simulink model "blovuztb"  (Simulink 8.5)
settings: Solver=ode45  SolverMode=SingleTasking  StartTime=0.0  StopTime=2  RelTol=1e-3  AbsTol=1e-6
settings Model: Creator=PC  LastModifiedBy=PC  ExtModeTrigMode=oneshot  ExtModeArmWhenConnect=off
settings DataIOCC: LimitDataPoints=off
settings OptimizationCC: BlockReduction=off  BooleanDataType=off  ExpressionDepthLimit=128
settings DebuggingCC: SaveWithParameterizedLinksMsg=none  SignalResolutionControl=TryResolveAllWithWarning  MultiTaskDSMMsg=warning  MultiTaskCondExecSysMsg=none  FcnCallInpInsideContextMsg=EnableAllAsError  StateNameClashWarn=none  StrictBusMsg=None
settings HardwareCC: TargetUnknown=on

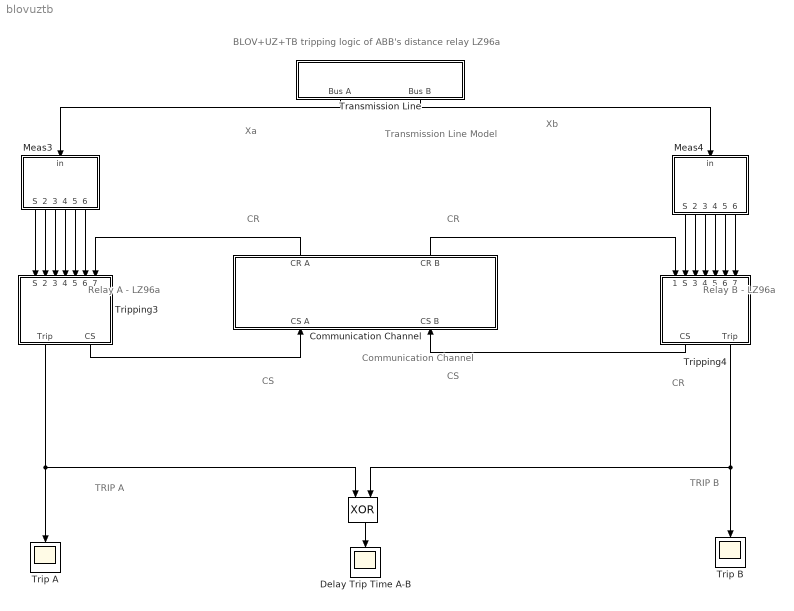
== system blovuztb ==
  note: Relay A - LZ96a
  note: CR
  note: Relay B - LZ96a
  note: Transmission Line Model
  note: Xa
  note: Xb
  note: CS
  note: CS
  note: CR
  note: CR
  note: BLOV+UZ+TB tripping logic of ABB's distance relay LZ96a
  note: Communication
      | Channel
  note: TRIP A
  note: TRIP B
  " " : Logic  Operator=XOR
  Communication Channel : Subsystem  mask(Communication channel.){Tdelay=20, failureA=off, failureB=on, err_signal=1}
      mask prompts: Tdelay "Channel delay time [ms]:"; failureA "A to B Communication channel failure."; failureB "B to A Communication Channel failure"; err_signal "Erroneous signal:"
      mask TypeOptions err_signal: 0 | 1
  Delay Trip Time A-B : Scope
      settings: TickLabels=on  YMin=-0.5  YMax=2
  Meas3 : Subsystem  mask(Tripping Logic){S=[3,1], ZM=[0.8, 1.6, 2.5], t=[0, 0.2, 0.4, 1], ZOV=[1.4, 0.02], ZMB=1.6}
      mask prompts: S "Starter  [Sfore(pu), Sback(pu)]:"; ZM "Zone reach [ZM1(pu), ZM2(pu), ZM3(pu)]:"; t "Zone time [t1(s), t2(s), t3(s), t4(s)] :"; ZOV "[ZOV(pu), tHF(s)] :"; ZMB "ZMB(pu):"
      mask help:
      | ABB LZ96a Distance Relay, BLOV+UZ+TB tripping logic :
      |    starters S (S, Ks, t4)
      |    measuring system M1 (ZM1, ZM2, ZM3), (0, t2, t3)
      |    measuring system M2 (ZOV, tHF)
      |    reverse measurement MB (ZMB)
      mask Help:
      | ABB LZ96a Distance Relay
      | BLOV+UZ+TB tripping logic
      | Blocking overreaching  with independent measuring zone and current reversal logic
  Meas4 : Subsystem  mask(Tripping Logic){S=[3,1], ZM=[0.8, 1.6, 2.5], t=[0, 0.2, 0.4, 1], ZOV=[1.4, 0.02], ZMB=1.6}
      mask prompts: S "Starter  [Sfore(pu), Sback(pu)]:"; ZM "Zone reach [ZM1(pu), ZM2(pu), ZM3(pu)]:"; t "Zone time [t1(s), t2(s), t3(s), t4(s)] :"; ZOV "[ZOV(pu), tHF(s)] :"; ZMB "ZMB(pu):"
      mask help:
      | ABB LZ96a Distance Relay, BLOV+UZ+TB tripping logic :
      |    starters S (S, Ks, t4)
      |    measuring system M1 (ZM1, ZM2, ZM3), (0, t2, t3)
      |    measuring system M2 (ZOV, tHF)
      |    reverse measurement MB (ZMB)
      mask Help:
      | ABB LZ96a Distance Relay
      | BLOV+UZ+TB tripping logic
      | Blocking overreaching  with independent measuring zone and current reversal logic
  Transmission Line : Subsystem  mask(Model of transmission line with fault){x=-0.1, Tfault=0}
      mask prompts: x "Fault location from bus A [p.u.]"; Tfault "Fault time [s]:"
  Trip A : Scope
      settings: TickLabels=on  TimeRange=2  YMin=-0.5  YMax=2
  Trip B : Scope
      settings: TickLabels=on  YMin=-0.5  YMax=2
  Tripping3 : Subsystem
  Tripping4 : Subsystem
  wires:
  Meas3/1(S) -> Tripping3/1(S)
  Meas3/2(ZM1) -> Tripping3/2(ZM1)
  Meas3/3(ZM2) -> Tripping3/3(ZM2)
  Meas3/4(ZM3) -> Tripping3/4(ZM3)
  Meas3/5(ZOV) -> Tripping3/5(ZOV)
  Meas3/6(ZMB) -> Tripping3/6(ZMB)
  Transmission Line/1(Bus A) -> Meas3/1(in)
  Communication Channel/1(CR A) -> Tripping3/7(CR)
  Tripping3/2(CS) -> Communication Channel/1(CS A)
  Meas4/1(S) -> Tripping4/2(S)
  Meas4/2(ZM1) -> Tripping4/3(ZM1)
  Meas4/3(ZM2) -> Tripping4/4(ZM2)
  Meas4/4(ZM3) -> Tripping4/5(ZM3)
  Meas4/5(ZOV) -> Tripping4/6(ZOV)
  Meas4/6(ZMB) -> Tripping4/7(ZMB)
  Transmission Line/2(Bus B) -> Meas4/1(in)
  Tripping4/1(CS) -> Communication Channel/2(CS B)
  Communication Channel/2(CR B) -> Tripping4/1(CR)
  " "/1 -> Delay Trip Time A-B/1
  Tripping3/1(Trip) -> Trip A/1, " "/1
  Tripping4/2(Trip) -> Trip B/1, " "/2

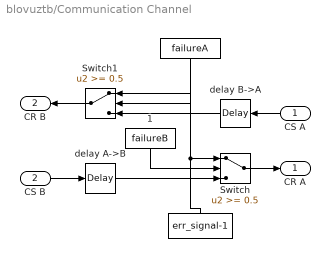
== system blovuztb/Communication Channel ==
  CS A : Inport
  CS B : Inport  Port=2
  " " : Constant  Value=failureA
  "  " : Constant  Value=err_signal-1
  " 1" : Constant  Value=failureB
  Switch : Switch  Threshold=0.5  SaturateOnIntegerOverflow=on  InputSameDT=on
  Switch1 : Switch  Threshold=0.5  SaturateOnIntegerOverflow=on  InputSameDT=on
  delay A->B : TransportDelay  DelayTime=Tdelay/1000+1e-12
  delay B->A : TransportDelay  DelayTime=Tdelay/1000+1e-12
  CR A : Outport  InitialOutput=0
  CR B : Outport  Port=2  InitialOutput=0
  wires:
  Switch/1 -> CR A/1
  CS B/1 -> delay A->B/1
  CS A/1 -> delay B->A/1
  Switch1/1 -> CR B/1
  "  "/1 -> Switch1/1, Switch/1
  delay A->B/1 -> Switch/3
  delay B->A/1 -> Switch1/3
  " "/1 -> Switch1/2
  " 1"/1 -> Switch/2

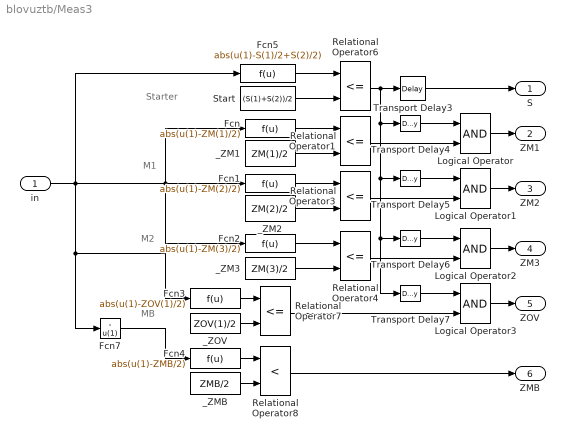
== system blovuztb/Meas3 ==
  note: M1
  note: Starter
  note: M2
  note: MB
  in : Inport
  Fcn : Fcn  Expr=abs(u(1)-ZM(1)/2)
  Fcn1 : Fcn  Expr=abs(u(1)-ZM(2)/2)
  Fcn2 : Fcn  Expr=abs(u(1)-ZM(3)/2)
  Fcn3 : Fcn  Expr=abs(u(1)-ZOV(1)/2)
  Fcn4 : Fcn  Expr=abs(u(1)-ZMB/2)
  Fcn5 : Fcn  Expr=abs(u(1)-S(1)/2+S(2)/2)
  Fcn7 : Fcn  Expr=- u(1)
  Logical Operator{,1..3} (4 alike) : Logic
  Relational Operator{1,3..4,6..7} (5 alike) : RelationalOperator  Operator=<=  InputSameDT=on
  Relational Operator8 : RelationalOperator  Operator=<  InputSameDT=on
  Start : Constant  Value=(S(1)+S(2))/2
  Transport Delay3 : TransportDelay  DelayTime=t(4)
  Transport Delay4 : TransportDelay  DelayTime=t(1)+1e-12
  Transport Delay5 : TransportDelay  DelayTime=t(2)
  Transport Delay6 : TransportDelay  DelayTime=t(3)
  Transport Delay7 : TransportDelay  DelayTime=ZOV(2)
  _ZM1 : Constant  Value=ZM(1)/2
  _ZM2 : Constant  Value=ZM(2)/2
  _ZM3 : Constant  Value=ZM(3)/2
  _ZMB : Constant  Value=ZMB/2
  _ZOV : Constant  Value=ZOV(1)/2
  S : Outport  InitialOutput=0
  ZM1 : Outport  Port=2  InitialOutput=0
  ZM2 : Outport  Port=3  InitialOutput=0
  ZM3 : Outport  Port=4  InitialOutput=0
  ZOV : Outport  Port=5  InitialOutput=0
  ZMB : Outport  Port=6  InitialOutput=0
  wires:
  _ZOV/1 -> Relational Operator7/2
  Fcn3/1 -> Relational Operator7/1
  _ZMB/1 -> Relational Operator8/2
  Fcn4/1 -> Relational Operator8/1
  in/1 -> Fcn5/1, Fcn3/1, Fcn7/1, Fcn1/1, Fcn/1, Fcn2/1
  _ZM1/1 -> Relational Operator1/2
  _ZM2/1 -> Relational Operator3/2
  Fcn1/1 -> Relational Operator3/1
  _ZM3/1 -> Relational Operator4/2
  Fcn2/1 -> Relational Operator4/1
  Start/1 -> Relational Operator6/2
  Fcn5/1 -> Relational Operator6/1
  Fcn/1 -> Relational Operator1/1
  Fcn7/1 -> Fcn4/1
  Relational Operator6/1 -> Transport Delay3/1, Transport Delay4/1, Transport Delay5/1, Transport Delay7/1, Transport Delay6/1
  Relational Operator8/1 -> ZMB/1
  Relational Operator1/1 -> Logical Operator/2
  Logical Operator/1 -> ZM1/1
  Transport Delay4/1 -> Logical Operator/1
  Relational Operator4/1 -> Logical Operator2/2
  Transport Delay6/1 -> Logical Operator2/1
  Logical Operator2/1 -> ZM3/1
  Relational Operator3/1 -> Logical Operator1/2
  Transport Delay5/1 -> Logical Operator1/1
  Logical Operator1/1 -> ZM2/1
  Transport Delay7/1 -> Logical Operator3/1
  Relational Operator7/1 -> Logical Operator3/2
  Logical Operator3/1 -> ZOV/1
  Transport Delay3/1 -> S/1

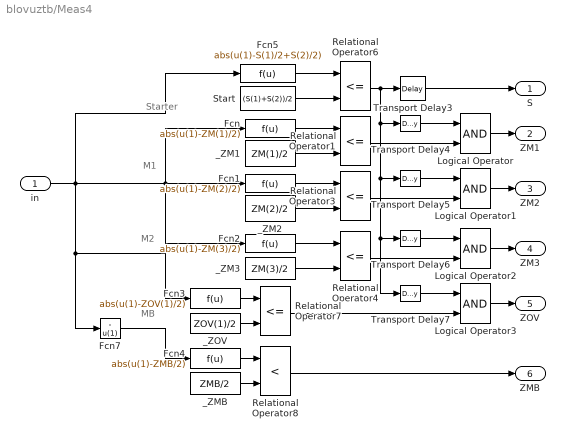
== system blovuztb/Meas4 ==
  note: MB
  note: M2
  note: Starter
  note: M1
  in : Inport
  Fcn : Fcn  Expr=abs(u(1)-ZM(1)/2)
  Fcn1 : Fcn  Expr=abs(u(1)-ZM(2)/2)
  Fcn2 : Fcn  Expr=abs(u(1)-ZM(3)/2)
  Fcn3 : Fcn  Expr=abs(u(1)-ZOV(1)/2)
  Fcn4 : Fcn  Expr=abs(u(1)-ZMB/2)
  Fcn5 : Fcn  Expr=abs(u(1)-S(1)/2+S(2)/2)
  Fcn7 : Fcn  Expr=- u(1)
  Logical Operator{,1..3} (4 alike) : Logic
  Relational Operator{1,3..4,6..7} (5 alike) : RelationalOperator  Operator=<=  InputSameDT=on
  Relational Operator8 : RelationalOperator  Operator=<  InputSameDT=on
  Start : Constant  Value=(S(1)+S(2))/2
  Transport Delay3 : TransportDelay  DelayTime=t(4)
  Transport Delay4 : TransportDelay  DelayTime=t(1)+1e-12
  Transport Delay5 : TransportDelay  DelayTime=t(2)
  Transport Delay6 : TransportDelay  DelayTime=t(3)
  Transport Delay7 : TransportDelay  DelayTime=ZOV(2)
  _ZM1 : Constant  Value=ZM(1)/2
  _ZM2 : Constant  Value=ZM(2)/2
  _ZM3 : Constant  Value=ZM(3)/2
  _ZMB : Constant  Value=ZMB/2
  _ZOV : Constant  Value=ZOV(1)/2
  S : Outport  InitialOutput=0
  ZM1 : Outport  Port=2  InitialOutput=0
  ZM2 : Outport  Port=3  InitialOutput=0
  ZM3 : Outport  Port=4  InitialOutput=0
  ZOV : Outport  Port=5  InitialOutput=0
  ZMB : Outport  Port=6  InitialOutput=0
  wires:
  Transport Delay3/1 -> S/1
  Logical Operator3/1 -> ZOV/1
  Relational Operator7/1 -> Logical Operator3/2
  Transport Delay7/1 -> Logical Operator3/1
  Logical Operator1/1 -> ZM2/1
  Transport Delay5/1 -> Logical Operator1/1
  Relational Operator3/1 -> Logical Operator1/2
  Logical Operator2/1 -> ZM3/1
  Transport Delay6/1 -> Logical Operator2/1
  Relational Operator4/1 -> Logical Operator2/2
  Transport Delay4/1 -> Logical Operator/1
  Logical Operator/1 -> ZM1/1
  Relational Operator1/1 -> Logical Operator/2
  Relational Operator8/1 -> ZMB/1
  Relational Operator6/1 -> Transport Delay6/1, Transport Delay7/1, Transport Delay5/1, Transport Delay4/1, Transport Delay3/1
  Fcn7/1 -> Fcn4/1
  Fcn/1 -> Relational Operator1/1
  Fcn5/1 -> Relational Operator6/1
  Start/1 -> Relational Operator6/2
  Fcn2/1 -> Relational Operator4/1
  _ZM3/1 -> Relational Operator4/2
  Fcn1/1 -> Relational Operator3/1
  _ZM2/1 -> Relational Operator3/2
  _ZM1/1 -> Relational Operator1/2
  in/1 -> Fcn2/1, Fcn/1, Fcn1/1, Fcn7/1, Fcn3/1, Fcn5/1
  Fcn4/1 -> Relational Operator8/1
  _ZMB/1 -> Relational Operator8/2
  Fcn3/1 -> Relational Operator7/1
  _ZOV/1 -> Relational Operator7/2

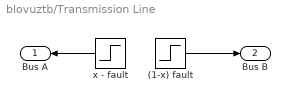
== system blovuztb/Transmission Line ==
  (1-x) fault : Step  Time=Tfault  Before=1000  After=1-x  SampleTime=0
  x - fault : Step  Time=Tfault  Before=1000  After=x  SampleTime=0
  Bus A : Outport  InitialOutput=0
  Bus B : Outport  Port=2  InitialOutput=0
  wires:
  (1-x) fault/1 -> Bus B/1
  x - fault/1 -> Bus A/1

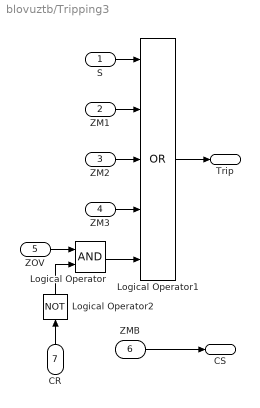
== system blovuztb/Tripping3 ==
  S : Inport
  ZM1 : Inport  Port=2
  ZM2 : Inport  Port=3
  ZM3 : Inport  Port=4
  ZOV : Inport  Port=5
  ZMB : Inport  Port=6
  CR : Inport  Port=7
  Logical Operator : Logic
  Logical Operator1 : Logic  Operator=OR  Inputs=5
  Logical Operator2 : Logic  Operator=NOT  Inputs=1
  Trip : Outport  InitialOutput=0
  CS : Outport  Port=2  InitialOutput=0
  wires:
  Logical Operator2/1 -> Logical Operator/2
  Logical Operator/1 -> Logical Operator1/5
  S/1 -> Logical Operator1/1
  ZM1/1 -> Logical Operator1/2
  ZM2/1 -> Logical Operator1/3
  ZM3/1 -> Logical Operator1/4
  ZOV/1 -> Logical Operator/1
  CR/1 -> Logical Operator2/1
  Logical Operator1/1 -> Trip/1
  ZMB/1 -> CS/1

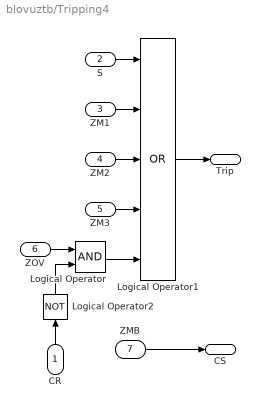
== system blovuztb/Tripping4 ==
  CR : Inport
  S : Inport  Port=2
  ZM1 : Inport  Port=3
  ZM2 : Inport  Port=4
  ZM3 : Inport  Port=5
  ZOV : Inport  Port=6
  ZMB : Inport  Port=7
  Logical Operator : Logic
  Logical Operator1 : Logic  Operator=OR  Inputs=5
  Logical Operator2 : Logic  Operator=NOT  Inputs=1
  CS : Outport  InitialOutput=0
  Trip : Outport  Port=2  InitialOutput=0
  wires:
  ZMB/1 -> CS/1
  Logical Operator1/1 -> Trip/1
  CR/1 -> Logical Operator2/1
  ZOV/1 -> Logical Operator/1
  ZM3/1 -> Logical Operator1/4
  ZM2/1 -> Logical Operator1/3
  ZM1/1 -> Logical Operator1/2
  S/1 -> Logical Operator1/1
  Logical Operator/1 -> Logical Operator1/5
  Logical Operator2/1 -> Logical Operator/2
